simulink model "sm_vehicle_slalom"  (R2021b)
settings: Solver=VariableStepAuto  StartTime=0.0  StopTime=25  MaxStep=0.01  RelTol=1e-3  EnableMultiTasking=on
model workspace: external: MATLAB File sm_vehicle_slalom_parameters.m (data not in the file)
undefined symbols (not defined in the file): filter, finishline, road, slalom, vehicle, X, Y, Z
libraries: sm_lib x45, sm_vehicle_slalom_lib x18, simulink x5, nesl_utility x4, fl_lib x3
(part 2 of 2)

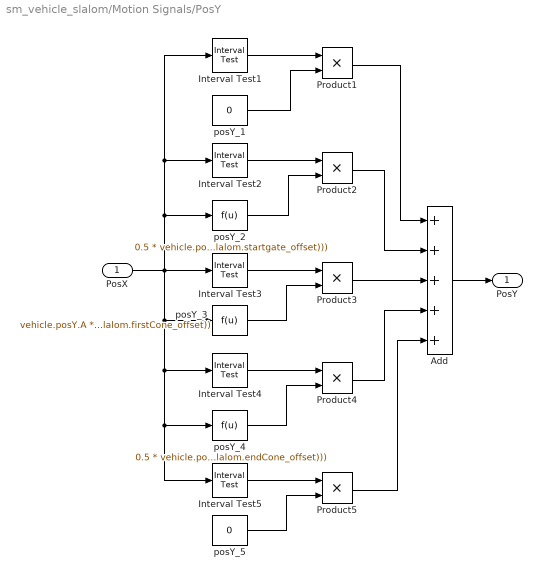
== system sm_vehicle_slalom/Motion Signals/PosY ==
  PosX : Inport
  Add : Sum  Inputs=+++++
  Interval Test1 : simulink/Logic and Bit Operations/Interval Test  IntervalClosedRight=on  uplimit=slalom.startgate_offset  IntervalClosedLeft=on  lowlimit=vehicle.posX_0  OutDataTypeStr=boolean
  Interval Test2 : simulink/Logic and Bit Operations/Interval Test  IntervalClosedRight=on  uplimit=slalom.firstCone_offset  IntervalClosedLeft=off  lowlimit=slalom.startgate_offset  OutDataTypeStr=boolean
  Interval Test3 : simulink/Logic and Bit Operations/Interval Test  IntervalClosedRight=on  uplimit=slalom.endCone_offset  IntervalClosedLeft=off  lowlimit=slalom.firstCone_offset  OutDataTypeStr=boolean
  Interval Test4 : simulink/Logic and Bit Operations/Interval Test  IntervalClosedRight=on  uplimit=slalom.finishgate_offset  IntervalClosedLeft=off  lowlimit=slalom.endCone_offset  OutDataTypeStr=boolean
  Interval Test5 : simulink/Logic and Bit Operations/Interval Test  IntervalClosedRight=on  uplimit=road.length  IntervalClosedLeft=off  lowlimit=slalom.finishgate_offset  OutDataTypeStr=boolean
  Product{1..5} (5 alike) : Product
  posY_1 : Constant  Value=0
  posY_2 : Fcn  Expr=0.5 * vehicle.posY.A * (1 - cos(pi / slalom.firstConeFromStartgate * (u - slalom.startgate_offset)))
  posY_3 : Fcn  Expr=vehicle.posY.A * cos(pi / slalom.coneSpacing * (u - slalom.firstCone_offset))
  posY_4 : Fcn  Expr=0.5 * vehicle.posY.A * (1 + cos(pi / (slalom.finishgateFromEndCone) * (u - slalom.endCone_offset)))
  posY_5 : Constant  Value=0
  PosY : Outport  VectorParamsAs1DForOutWhenUnconnected=off
  wires:
  Add/1 -> PosY/1
  PosX/1 -> Interval Test5/1, posY_4/1, Interval Test4/1, posY_3/1, Interval Test1/1, Interval Test2/1, posY_2/1, Interval Test3/1
  posY_1/1 -> Product1/2
  Interval Test1/1 -> Product1/1
  Interval Test2/1 -> Product2/1
  posY_2/1 -> Product2/2
  posY_3/1 -> Product3/2
  Interval Test3/1 -> Product3/1
  Interval Test4/1 -> Product4/1
  posY_4/1 -> Product4/2
  Interval Test5/1 -> Product5/1
  posY_5/1 -> Product5/2
  Product3/1 -> Add/3
  Product2/1 -> Add/2
  Product1/1 -> Add/1
  Product4/1 -> Add/4
  Product5/1 -> Add/5

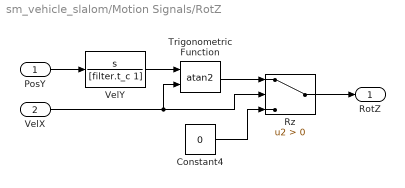
== system sm_vehicle_slalom/Motion Signals/RotZ ==
  PosY : Inport
  VelX : Inport  Port=2
  Constant4 : Constant  Value=0
  Rz : Switch  Criteria=u2 > Threshold
  Trigonometric Function : Trigonometry  Operator=atan2
  VelY : TransferFcn  Numerator=[1 0]  Denominator=[filter.t_c 1]
  RotZ : Outport  VectorParamsAs1DForOutWhenUnconnected=off
  wires:
  PosY/1 -> VelY/1
  VelY/1 -> Trigonometric Function/1
  Rz/1 -> RotZ/1
  Trigonometric Function/1 -> Rz/1
  Constant4/1 -> Rz/3
  VelX/1 -> Rz/2, Trigonometric Function/2

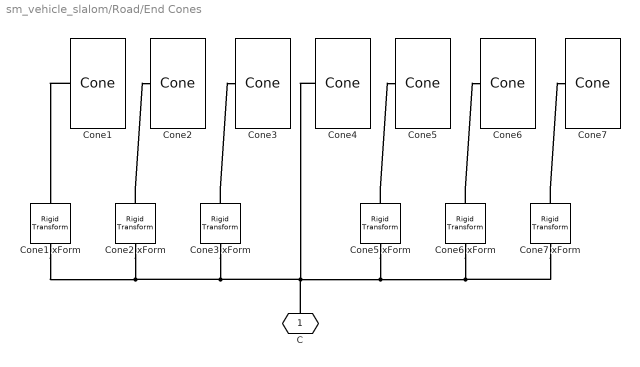
== system sm_vehicle_slalom/Road/End Cones ==
  Cone{1..7} (7 alike) : sm_vehicle_slalom_lib/Cone  height=tallCone.height  baseThickness=tallCone.baseThickness  baseDiameter=tallCone.baseDiameter  coneBaseDiameter=tallCone.coneBaseDiameter  coneTopDiameter=tallCone.coneTopDiameter  reflectiveStripHeight=tallCone.reflectiveStripHeight  coneColor=tallCone.coneColor  reflectiveStripColor=tallCone.reflectiveStripColor
      settings: SourceProductBaseCode=MS
  Cone1 xForm : sm_lib/Frames and Transforms/Rigid Transform  TranslationMethod=StandardAxis  TranslationStandardOffset=3 * finishline.cones.spacing  TranslationLengthUnit=m  TranslationStandardAxis=+Y  TranslationCartesianOffset=[0 0 0]  TranslationROffset=0  TranslationROffsetUnits=m  TranslationZOffset=0  TranslationZOffsetUnits=m  TranslationThetaOffset=0  TranslationThetaOffsetUnits=deg  RotationMethod=None  RotationAngleUnits=deg  RotationStandardAxis=+Z  RotationAngle=0.0  RotationArbitraryAxis=[0 0 1]  FollAlignAxisA=+X  BaseAlignAxisA=+Y  FollAlignAxisB=+Y  BaseAlignAxisB=+Z  RotationSequenceAxes=FollowerAxes  RotationSequence=XYX  RotationSequenceAngles=[0 0 0]  RotationSequenceAnglesUnits=deg  RotationMatrix=[1 0 0; 0 1 0; 0 0 1]
  Cone2 xForm : sm_lib/Frames and Transforms/Rigid Transform  TranslationMethod=StandardAxis  TranslationStandardOffset=2 * finishline.cones.spacing  TranslationLengthUnit=m  TranslationStandardAxis=+Y  TranslationCartesianOffset=[0 0 0]  TranslationROffset=0  TranslationROffsetUnits=m  TranslationZOffset=0  TranslationZOffsetUnits=m  TranslationThetaOffset=0  TranslationThetaOffsetUnits=deg  RotationMethod=None  RotationAngleUnits=deg  RotationStandardAxis=+Z  RotationAngle=0.0  RotationArbitraryAxis=[0 0 1]  FollAlignAxisA=+X  BaseAlignAxisA=+Y  FollAlignAxisB=+Y  BaseAlignAxisB=+Z  RotationSequenceAxes=FollowerAxes  RotationSequence=XYX  RotationSequenceAngles=[0 0 0]  RotationSequenceAnglesUnits=deg  RotationMatrix=[1 0 0; 0 1 0; 0 0 1]
  Cone3 xForm : sm_lib/Frames and Transforms/Rigid Transform  TranslationMethod=StandardAxis  TranslationStandardOffset=finishline.cones.spacing  TranslationLengthUnit=m  TranslationStandardAxis=+Y  TranslationCartesianOffset=[0 0 0]  TranslationROffset=0  TranslationROffsetUnits=m  TranslationZOffset=0  TranslationZOffsetUnits=m  TranslationThetaOffset=0  TranslationThetaOffsetUnits=deg  RotationMethod=None  RotationAngleUnits=deg  RotationStandardAxis=+Z  RotationAngle=0.0  RotationArbitraryAxis=[0 0 1]  FollAlignAxisA=+X  BaseAlignAxisA=+Y  FollAlignAxisB=+Y  BaseAlignAxisB=+Z  RotationSequenceAxes=FollowerAxes  RotationSequence=XYX  RotationSequenceAngles=[0 0 0]  RotationSequenceAnglesUnits=deg  RotationMatrix=[1 0 0; 0 1 0; 0 0 1]
  Cone5 xForm : sm_lib/Frames and Transforms/Rigid Transform  TranslationMethod=StandardAxis  TranslationStandardOffset=finishline.cones.spacing  TranslationLengthUnit=m  TranslationStandardAxis=-Y  TranslationCartesianOffset=[0 0 0]  TranslationROffset=0  TranslationROffsetUnits=m  TranslationZOffset=0  TranslationZOffsetUnits=m  TranslationThetaOffset=0  TranslationThetaOffsetUnits=deg  RotationMethod=None  RotationAngleUnits=deg  RotationStandardAxis=+Z  RotationAngle=0.0  RotationArbitraryAxis=[0 0 1]  FollAlignAxisA=+X  BaseAlignAxisA=+Y  FollAlignAxisB=+Y  BaseAlignAxisB=+Z  RotationSequenceAxes=FollowerAxes  RotationSequence=XYX  RotationSequenceAngles=[0 0 0]  RotationSequenceAnglesUnits=deg  RotationMatrix=[1 0 0; 0 1 0; 0 0 1]
  Cone6 xForm : sm_lib/Frames and Transforms/Rigid Transform  TranslationMethod=StandardAxis  TranslationStandardOffset=2 * finishline.cones.spacing  TranslationLengthUnit=m  TranslationStandardAxis=-Y  TranslationCartesianOffset=[0 0 0]  TranslationROffset=0  TranslationROffsetUnits=m  TranslationZOffset=0  TranslationZOffsetUnits=m  TranslationThetaOffset=0  TranslationThetaOffsetUnits=deg  RotationMethod=None  RotationAngleUnits=deg  RotationStandardAxis=+Z  RotationAngle=0.0  RotationArbitraryAxis=[0 0 1]  FollAlignAxisA=+X  BaseAlignAxisA=+Y  FollAlignAxisB=+Y  BaseAlignAxisB=+Z  RotationSequenceAxes=FollowerAxes  RotationSequence=XYX  RotationSequenceAngles=[0 0 0]  RotationSequenceAnglesUnits=deg  RotationMatrix=[1 0 0; 0 1 0; 0 0 1]
  Cone7 xForm : sm_lib/Frames and Transforms/Rigid Transform  TranslationMethod=StandardAxis  TranslationStandardOffset=3 * finishline.cones.spacing  TranslationLengthUnit=m  TranslationStandardAxis=-Y  TranslationCartesianOffset=[0 0 0]  TranslationROffset=0  TranslationROffsetUnits=m  TranslationZOffset=0  TranslationZOffsetUnits=m  TranslationThetaOffset=0  TranslationThetaOffsetUnits=deg  RotationMethod=None  RotationAngleUnits=deg  RotationStandardAxis=+Z  RotationAngle=0.0  RotationArbitraryAxis=[0 0 1]  FollAlignAxisA=+X  BaseAlignAxisA=+Y  FollAlignAxisB=+Y  BaseAlignAxisB=+Z  RotationSequenceAxes=FollowerAxes  RotationSequence=XYX  RotationSequenceAngles=[0 0 0]  RotationSequenceAnglesUnits=deg  RotationMatrix=[1 0 0; 0 1 0; 0 0 1]
  C : PMIOPort  Side=Left
  connections:
  Cone4/LConn1 -- Cone1 xForm/LConn1 -- Cone2 xForm/LConn1 -- Cone3 xForm/LConn1 -- C/RConn1 -- Cone7 xForm/LConn1 -- Cone6 xForm/LConn1 -- Cone5 xForm/LConn1
  Cone1/LConn1 -- Cone1 xForm/RConn1
  Cone2 xForm/RConn1 -- Cone2/LConn1
  Cone3 xForm/RConn1 -- Cone3/LConn1
  Cone5 xForm/RConn1 -- Cone5/LConn1
  Cone6 xForm/RConn1 -- Cone6/LConn1
  Cone7 xForm/RConn1 -- Cone7/LConn1

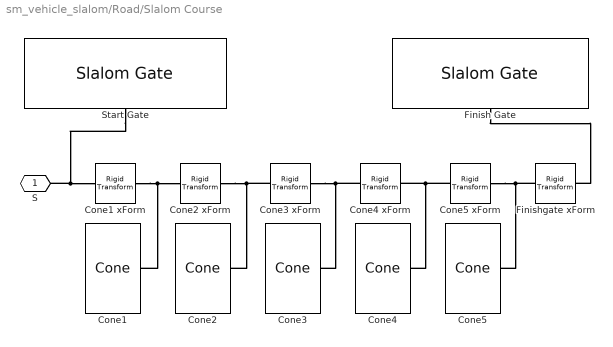
== system sm_vehicle_slalom/Road/Slalom Course ==
  Cone{1..5} (5 alike) : sm_vehicle_slalom_lib/Cone  height=shortCone.height  baseThickness=shortCone.baseThickness  baseDiameter=shortCone.baseDiameter  coneBaseDiameter=shortCone.coneBaseDiameter  coneTopDiameter=shortCone.coneTopDiameter  reflectiveStripHeight=shortCone.reflectiveStripHeight  coneColor=shortCone.coneColor  reflectiveStripColor=shortCone.reflectiveStripColor
      settings: SourceProductBaseCode=MS
  Cone1 xForm : sm_lib/Frames and Transforms/Rigid Transform  TranslationMethod=StandardAxis  TranslationStandardOffset=slalom.firstConeFromStartgate  TranslationLengthUnit=m  TranslationStandardAxis=+X  TranslationCartesianOffset=[0 0 0]  TranslationROffset=0  TranslationROffsetUnits=m  TranslationZOffset=0  TranslationZOffsetUnits=m  TranslationThetaOffset=0  TranslationThetaOffsetUnits=deg  RotationMethod=None  RotationAngleUnits=deg  RotationStandardAxis=+Z  RotationAngle=0.0  RotationArbitraryAxis=[0 0 1]  FollAlignAxisA=+X  BaseAlignAxisA=+Y  FollAlignAxisB=+Y  BaseAlignAxisB=+Z  RotationSequenceAxes=FollowerAxes  RotationSequence=XYX  RotationSequenceAngles=[0 0 0]  RotationSequenceAnglesUnits=deg  RotationMatrix=[1 0 0; 0 1 0; 0 0 1]
  Cone2 xForm : sm_lib/Frames and Transforms/Rigid Transform  TranslationMethod=StandardAxis  TranslationStandardOffset=slalom.coneSpacing  TranslationLengthUnit=m  TranslationStandardAxis=+X  TranslationCartesianOffset=[0 0 0]  TranslationROffset=0  TranslationROffsetUnits=m  TranslationZOffset=0  TranslationZOffsetUnits=m  TranslationThetaOffset=0  TranslationThetaOffsetUnits=deg  RotationMethod=None  RotationAngleUnits=deg  RotationStandardAxis=+Z  RotationAngle=0.0  RotationArbitraryAxis=[0 0 1]  FollAlignAxisA=+X  BaseAlignAxisA=+Y  FollAlignAxisB=+Y  BaseAlignAxisB=+Z  RotationSequenceAxes=FollowerAxes  RotationSequence=XYX  RotationSequenceAngles=[0 0 0]  RotationSequenceAnglesUnits=deg  RotationMatrix=[1 0 0; 0 1 0; 0 0 1]
  Cone3 xForm : sm_lib/Frames and Transforms/Rigid Transform  TranslationMethod=StandardAxis  TranslationStandardOffset=slalom.coneSpacing  TranslationLengthUnit=m  TranslationStandardAxis=+X  TranslationCartesianOffset=[0 0 0]  TranslationROffset=0  TranslationROffsetUnits=m  TranslationZOffset=0  TranslationZOffsetUnits=m  TranslationThetaOffset=0  TranslationThetaOffsetUnits=deg  RotationMethod=None  RotationAngleUnits=deg  RotationStandardAxis=+Z  RotationAngle=0.0  RotationArbitraryAxis=[0 0 1]  FollAlignAxisA=+X  BaseAlignAxisA=+Y  FollAlignAxisB=+Y  BaseAlignAxisB=+Z  RotationSequenceAxes=FollowerAxes  RotationSequence=XYX  RotationSequenceAngles=[0 0 0]  RotationSequenceAnglesUnits=deg  RotationMatrix=[1 0 0; 0 1 0; 0 0 1]
  Cone4 xForm : sm_lib/Frames and Transforms/Rigid Transform  TranslationMethod=StandardAxis  TranslationStandardOffset=slalom.coneSpacing  TranslationLengthUnit=m  TranslationStandardAxis=+X  TranslationCartesianOffset=[0 0 0]  TranslationROffset=0  TranslationROffsetUnits=m  TranslationZOffset=0  TranslationZOffsetUnits=m  TranslationThetaOffset=0  TranslationThetaOffsetUnits=deg  RotationMethod=None  RotationAngleUnits=deg  RotationStandardAxis=+Z  RotationAngle=0.0  RotationArbitraryAxis=[0 0 1]  FollAlignAxisA=+X  BaseAlignAxisA=+Y  FollAlignAxisB=+Y  BaseAlignAxisB=+Z  RotationSequenceAxes=FollowerAxes  RotationSequence=XYX  RotationSequenceAngles=[0 0 0]  RotationSequenceAnglesUnits=deg  RotationMatrix=[1 0 0; 0 1 0; 0 0 1]
  Cone5 xForm : sm_lib/Frames and Transforms/Rigid Transform  TranslationMethod=StandardAxis  TranslationStandardOffset=slalom.coneSpacing  TranslationLengthUnit=m  TranslationStandardAxis=+X  TranslationCartesianOffset=[0 0 0]  TranslationROffset=0  TranslationROffsetUnits=m  TranslationZOffset=0  TranslationZOffsetUnits=m  TranslationThetaOffset=0  TranslationThetaOffsetUnits=deg  RotationMethod=None  RotationAngleUnits=deg  RotationStandardAxis=+Z  RotationAngle=0.0  RotationArbitraryAxis=[0 0 1]  FollAlignAxisA=+X  BaseAlignAxisA=+Y  FollAlignAxisB=+Y  BaseAlignAxisB=+Z  RotationSequenceAxes=FollowerAxes  RotationSequence=XYX  RotationSequenceAngles=[0 0 0]  RotationSequenceAnglesUnits=deg  RotationMatrix=[1 0 0; 0 1 0; 0 0 1]
  Finish Gate : sm_vehicle_slalom_lib/Slalom Gate  offset=slalom.gate.cone_offset  height=tallCone.height  baseThickness=tallCone.baseThickness  baseDiameter=tallCone.baseDiameter  coneBaseDiameter=tallCone.coneBaseDiameter  coneTopDiameter=tallCone.coneTopDiameter  reflectiveStripHeight=tallCone.reflectiveStripHeight  coneColor=tallCone.coneColor  reflectiveStripColor=tallCone.reflectiveStripColor
      settings: SourceProductBaseCode=MS
  Finishgate xForm : sm_lib/Frames and Transforms/Rigid Transform  TranslationMethod=StandardAxis  TranslationStandardOffset=slalom.finishgateFromEndCone  TranslationLengthUnit=m  TranslationStandardAxis=+X  TranslationCartesianOffset=[0 0 0]  TranslationROffset=0  TranslationROffsetUnits=m  TranslationZOffset=0  TranslationZOffsetUnits=m  TranslationThetaOffset=0  TranslationThetaOffsetUnits=deg  RotationMethod=None  RotationAngleUnits=deg  RotationStandardAxis=+Z  RotationAngle=0.0  RotationArbitraryAxis=[0 0 1]  FollAlignAxisA=+X  BaseAlignAxisA=+Y  FollAlignAxisB=+Y  BaseAlignAxisB=+Z  RotationSequenceAxes=FollowerAxes  RotationSequence=XYX  RotationSequenceAngles=[0 0 0]  RotationSequenceAnglesUnits=deg  RotationMatrix=[1 0 0; 0 1 0; 0 0 1]
  Start Gate : sm_vehicle_slalom_lib/Slalom Gate  offset=slalom.gate.cone_offset  height=tallCone.height  baseThickness=tallCone.baseThickness  baseDiameter=tallCone.baseDiameter  coneBaseDiameter=tallCone.coneBaseDiameter  coneTopDiameter=tallCone.coneTopDiameter  reflectiveStripHeight=tallCone.reflectiveStripHeight  coneColor=tallCone.coneColor  reflectiveStripColor=tallCone.reflectiveStripColor
      settings: SourceProductBaseCode=MS
  S : PMIOPort  Side=Left
  connections:
  Finish Gate/LConn1 -- Finishgate xForm/RConn1
  Start Gate/LConn1 -- Cone1 xForm/LConn1 -- S/RConn1
  Cone5 xForm/RConn1 -- Finishgate xForm/LConn1 -- Cone5/LConn1
  Cone5 xForm/LConn1 -- Cone4/LConn1 -- Cone4 xForm/RConn1
  Cone3 xForm/RConn1 -- Cone4 xForm/LConn1 -- Cone3/LConn1
  Cone2 xForm/RConn1 -- Cone3 xForm/LConn1 -- Cone2/LConn1
  Cone1 xForm/RConn1 -- Cone1/LConn1 -- Cone2 xForm/LConn1

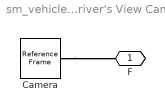
== system sm_vehicle_slalom/Vehicle/Driver's View Cam ==
  Camera : sm_lib/Frames and Transforms/Reference Frame
  F : PMIOPort  Side=Right
  connections:
  Camera/RConn1 -- F/RConn1
